simulink model "prog_controlwhat"  (R2024a)
settings: Solver=VariableStepAuto  StartTime=0.0  StopTime=4*pi  RelTol=1e-3
settings Model: Creator=Lisa  LastModifiedBy=pupkinzalupkin
settings OptimizationCC: ReuseModelBlockBuffer=off
settings RTWCC: GPUComputeCapability=3.5

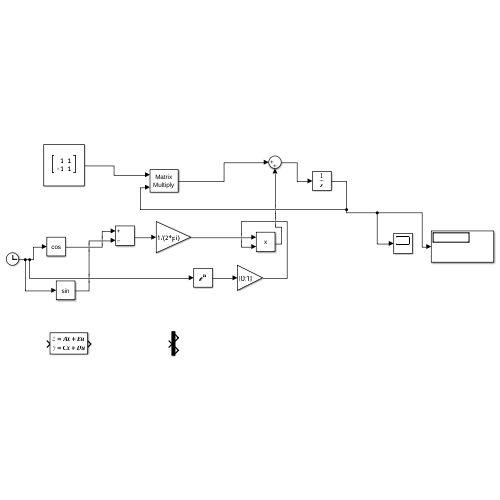
[thumbnail: Simulink's stored preview of the top-level diagram]
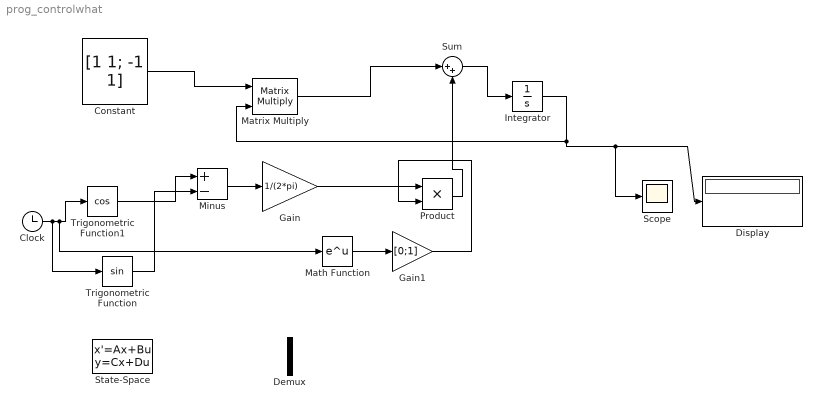
== system prog_controlwhat ==
  Clock : Clock
  Constant : Constant  Value=[1 1; -1 1]
  Demux : Demux  Outputs=2
  Display : Display
  Gain : Gain  Gain=1/(2*pi)
  Gain1 : Gain  Gain=[0;1]
  Integrator : Integrator  InitialCondition=[-1;-1]
  Math Function : Math
  Matrix Multiply : Product  Multiplication=Matrix(*)
  Minus : Sum  Inputs=+-
  Product : Product
  Scope : Scope
  State-Space : StateSpace  InitialCondition=0
  Sum : Sum  Inputs=|++
  Trigonometric Function : Trigonometry
  Trigonometric Function1 : Trigonometry  Operator=cos
  wires:
  Trigonometric Function1/1 -> Minus/1
  Trigonometric Function/1 -> Minus/2
  Minus/1 -> Gain/1
  Clock/1 -> Trigonometric Function/1, Math Function/1, Trigonometric Function1/1
  Integrator/1 -> Scope/1, Display/1, Matrix Multiply/2
  Math Function/1 -> Gain1/1
  Constant/1 -> Matrix Multiply/1
  Gain/1 -> Product/1
  Product/1 -> Sum/2
  Gain1/1 -> Product/2
  Matrix Multiply/1 -> Sum/1
  Sum/1 -> Integrator/1
